simulink model "circle"  (Simulink 7.3)
settings: Solver=ode3  StartTime=0.0  StopTime=1000  FixedStep=1  RelTol=1e-3
undefined symbols (not defined in the file): DiscIntNeverNeededParam
libraries: simulink x1
settings Model: Creator=Natalia  LastModifiedBy=Natalia

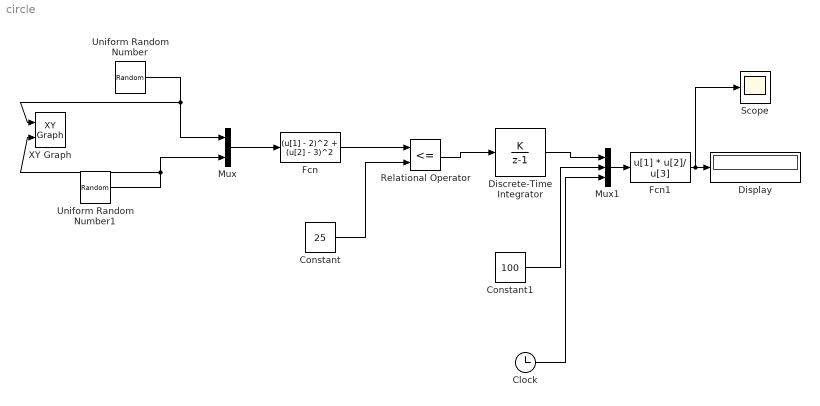
== system circle ==
  Clock : Clock
      settings: Decimation=10
  Constant : Constant  Value=25  OutDataType=fixdt(1, 16)  OutScaling=2^0
  Constant1 : Constant  Value=100  OutDataType=fixdt(1, 16)  OutScaling=2^0
  Discrete-Time Integrator : DiscreteIntegrator  IntegratorMethod=Accumulation: Forward Euler  gainval=1  OutDataTypeMode=double  OutDataType=fixdt(1, 16)  OutScaling=2^0  OutDataTypeStr=double  ICPrevOutput=DiscIntNeverNeededParam  ICPrevScaledInput=DiscIntNeverNeededParam
  Display : Display
  Fcn : Fcn  Expr=(u[1] - 2)^2 + (u[2] - 3)^2
  Fcn1 : Fcn  Expr=u[1] * u[2]/ u[3]
  Mux : Mux  Inputs=2
  Mux1 : Mux  Inputs=3
  Relational Operator : RelationalOperator  Operator=<=  LogicOutDataTypeMode=boolean  LogicDataType=fixdt(0, 8)  OutDataTypeStr=boolean
  Scope : Scope
  Uniform Random Number : UniformRandomNumber  Minimum=-3  SampleTime=0
  Uniform Random Number1 : UniformRandomNumber  Minimum=-2  Maximum=8  Seed=7  SampleTime=0
  XY Graph : simulink/Sinks/XY Graph  SystemSampleTime=-1  xmin=-1  xmax=1  ymin=-1  ymax=1  st=-1
  wires:
  Uniform Random Number/1 -> Mux/1, XY Graph/1
  Uniform Random Number1/1 -> Mux/2, XY Graph/2
  Mux/1 -> Fcn/1
  Fcn/1 -> Relational Operator/1
  Constant/1 -> Relational Operator/2
  Relational Operator/1 -> Discrete-Time Integrator/1
  Discrete-Time Integrator/1 -> Mux1/1
  Constant1/1 -> Mux1/2
  Clock/1 -> Mux1/3
  Mux1/1 -> Fcn1/1
  Fcn1/1 -> Display/1, Scope/1
